simulink model "OA_Dynamic"  (R2020a)
settings: Solver=VariableStepAuto  StartTime=0.0  StopTime=30  RelTol=1e-3
values from neighbouring files (symbols this model uses):
  b = 0.4    [Takeoff.m]
  body_rate_0 = [0;0;0]    [Takeoff.m]
  Boundaries = [B1;B2;B3]    [Takeoff.m]
  Euler_0 = [0;0;0]    [Takeoff.m]
  g = [0;0;-9.8]    [Takeoff.m]
  I_Drone = [0.3933,0.3933,0.76]    [Takeoff.m]
  I_Tank = CalItank(m_tank,0.4,0.1,0.4,i)    [Takeoff.m]
  J = 0.00062    [Takeoff.m]
  K = 0.074    [Takeoff.m]
  k_T = MaxMotorThrsut/(MaxRPM^2)    (= 6.99167657551e-06)    [Takeoff.m]
  k_Thrsut2Torque = 0.021    [Takeoff.m]
  l = 0.5    [Takeoff.m]
  L = sqrt((x2-x1)^2 + (y2-y1)^2)    [Takeoff.m]
  m = m_drone + m_tank*percent    (= 36)    [Takeoff.m]    (also in animation.m = T_V1toI*T_V2toV1*T_BtoV2)
  m_drone = 20    [Takeoff.m]
  m_tank = 16    [Takeoff.m]
  MaxThrust = 4*MaxMotorThrsut    (= 529.2)    [Takeoff.m]
  MaxTilt = 30*pi/180    (= 0.523598775598)    [Takeoff.m]
  MaxTorque_XY = (T2-T1)*(l/sqrt(2))    [Takeoff.m]
  MaxVolt = 48    [Takeoff.m]
  MaxYawRate = 100*pi/180    (= 1.74532925199)    [Takeoff.m]
  MaxZVel = 2    [Takeoff.m]
  percent = 1    [Takeoff.m]
  Px1 = 0.2    [Takeoff.m]
  Pz1 = 1    [Takeoff.m]
  Pz2 = 100    [Takeoff.m]
  R = 0.0062    [Takeoff.m]
  RecObstacle = [[5,4,3] ... (first row only)    [Takeoff.m]
  SafeZone = 1.0    (= 1)    [Takeoff.m]
  Target = WayPts(3,:)    [Takeoff.m]
  ts = 0.01    [Takeoff.m]
  WayPts = [[XYZ_0(1) XYZ_0(2) XYZ_0(3)] ... (first row only)    [Takeoff.m]
  XYZ_0 = [0;0;0]    [Takeoff.m]
undefined symbols (not defined in the file or in its folder): b_tank, d_drone, d_tank, DiscIntNeverNeededParam, FlyVel, h_tank, PD1, PD2, PI1, PI2, PP1, PP2, SafeFactor, Sensor0Dir, TestVel
libraries: simulink x27, vrlib x4
(part 3 of 3)

== system OA_Dynamic/Controller/Rotors System/Propellers/Motor Thrust Control1/DC Motor ==
  note: d2/dt2(theta)
  note: d/dt(theta)
  note: d/dt(i)
  note: i
  Voltage : Inport
  TQ_load : Inport  Port=2
  Add : Sum  Inputs=-+-
  Add1 : Sum  Inputs=+--
  Damping : Gain  Gain=b
  Inductance : Gain  Gain=1/L
  Inertia : Gain  Gain=1/J
  Integrator : Integrator
  Integrator1 : Integrator
  Ke : Gain  Gain=K
  Kt : Gain  Gain=K
  Resistance : Gain  Gain=R
  Scope : Scope  NumInputPorts=2
  Speed : Outport
  wires:
  TQ_load/1 -> Add1/3
  Add1/1 -> Inertia/1
  Add/1 -> Inductance/1
  Ke/1 -> Add/3
  Damping/1 -> Add1/2
  Resistance/1 -> Add/1
  Voltage/1 -> Add/2
  Kt/1 -> Add1/1
  Integrator/1 -> Resistance/1, Scope/1, Kt/1
  Inertia/1 -> Integrator1/1
  Integrator1/1 -> Ke/1, Speed/1, Scope/2, Damping/1
  Inductance/1 -> Integrator/1

== system OA_Dynamic/Controller/Rotors System/Propellers/Motor Thrust Control2/DC Motor ==
  note: i
  note: d/dt(i)
  note: d/dt(theta)
  note: d2/dt2(theta)
  Voltage : Inport
  TQ_load : Inport  Port=2
  Add : Sum  Inputs=-+-
  Add1 : Sum  Inputs=+--
  Damping : Gain  Gain=b
  Inductance : Gain  Gain=1/L
  Inertia : Gain  Gain=1/J
  Integrator : Integrator
  Integrator1 : Integrator
  Ke : Gain  Gain=K
  Kt : Gain  Gain=K
  Resistance : Gain  Gain=R
  Scope : Scope  NumInputPorts=2
  Speed : Outport
  wires:
  Inductance/1 -> Integrator/1
  Integrator1/1 -> Damping/1, Scope/2, Speed/1, Ke/1
  Inertia/1 -> Integrator1/1
  Integrator/1 -> Kt/1, Scope/1, Resistance/1
  Kt/1 -> Add1/1
  Voltage/1 -> Add/2
  Resistance/1 -> Add/1
  Damping/1 -> Add1/2
  Ke/1 -> Add/3
  Add/1 -> Inductance/1
  Add1/1 -> Inertia/1
  TQ_load/1 -> Add1/3

== system OA_Dynamic/Controller/Rotors System/Propellers/Motor Thrust Control3/DC Motor ==
  note: d2/dt2(theta)
  note: d/dt(theta)
  note: d/dt(i)
  note: i
  Voltage : Inport
  TQ_load : Inport  Port=2
  Add : Sum  Inputs=-+-
  Add1 : Sum  Inputs=+--
  Damping : Gain  Gain=b
  Inductance : Gain  Gain=1/L
  Inertia : Gain  Gain=1/J
  Integrator : Integrator
  Integrator1 : Integrator
  Ke : Gain  Gain=K
  Kt : Gain  Gain=K
  Resistance : Gain  Gain=R
  Scope : Scope  NumInputPorts=2
  Speed : Outport
  wires:
  TQ_load/1 -> Add1/3
  Add1/1 -> Inertia/1
  Add/1 -> Inductance/1
  Ke/1 -> Add/3
  Damping/1 -> Add1/2
  Resistance/1 -> Add/1
  Voltage/1 -> Add/2
  Kt/1 -> Add1/1
  Integrator/1 -> Resistance/1, Scope/1, Kt/1
  Inertia/1 -> Integrator1/1
  Integrator1/1 -> Ke/1, Speed/1, Scope/2, Damping/1
  Inductance/1 -> Integrator/1

== matlab function OA_Dynamic/Controller/Sense X Y Distance/Sensor0 (30 degree sensor) ==
  data: Pos input; MinBDist output; Bounds input; Yaw input; MinBVect output; Directions input
function [MinBDist,MinBVect] = fcn(Pos,Bounds,Yaw,Directions)
MinBDist = 999;
MinBVect = [1;0;0];

for b = 1:size(Bounds,1)
Bound = Bounds(b,:);

%Bound = Bounds(BIndex,:);
MinSenseDist = 999;
MinSenseVect = [1;0;0];

for k = 1:size(Directions,2)
if length(Pos) > 1
    bx = Bound(1);
    by = Bound(2);
    tx = Bound(3);
    ty = Bound(4);
    X = Pos(1);
    Y = Pos(2);
    Z = Pos(3);
    
    m = [[cos(Yaw) -sin(Yaw)];[sin(Yaw) cos(Yaw)]];
    n = m*Directions(:,k); % Sense vector
    nx = n(1);
    ny = n(2);

    j = ((ty*bx-tx*by)-(ty*X-tx*Y))/(ty*nx-tx*ny);
    
    if j < 0 % sense backward point
        SenseDist = 999;
    else
        SensePt = [X+nx*j;Y+ny*j];
        
        % Check if ON boundaries
        if tx == 0
            i = (SensePt(2)-by)/ty;
        else
            i = (SensePt(1)-bx)/tx;
        end
        
        % If not
        if i < 0 || i > Bound(7)
            SenseDist = 999;
        % If yes
        else
            SenseDist = sqrt((nx*j)^2 + (ny*j)^2);
        end
    end
    
    SenseVect = [nx;ny;0]/sqrt(nx^2+ny^2);
    
else
    SenseDist = 999;
    SenseVect = [0;0;0];
end


if SenseDist < MinSenseDist
    MinSenseDist = SenseDist;
    MinSenseVect = SenseVect;
end
end

if MinSenseDist < MinBDist
    MinBDist = MinSenseDist;
    MinBVect = MinSenseVect;
end
end

== matlab function OA_Dynamic/6dof_system/Drone & Liquid Dynamic Inertia/DroneTankI ==
  data: I_D input; I output; I_T input; M_D input; M_T input; Z_D input; Z_T input; CR_X input; CR_Y input
function I = fcn(I_D,I_T,M_D,M_T,Z_D,Z_T,CR_X,CR_Y)

    Ix = I_D(1) + M_D*Z_D^2 + CR_X*I_T(1) + M_T*Z_T^2;
    Iy = I_D(2) + M_D*Z_D^2 + CR_Y*I_T(2) + M_T*Z_T^2;
    Iz = I_D(3) + I_T(3);
    I = [[Ix 0 0];[0 Iy 0];[0 0 Iz]];

== matlab function OA_Dynamic/6dof_system/Drone & Liquid Dynamic Inertia/FullTankCR ==
  data: w_d input; CR_x output; CR_y output; C_R input
function [CR_x,CR_y] = fcn(w_d,C_R)
if length(w_d) > 1
    if abs(w_d(2)) > 0.001
        CR_y = C_R;
    else
        CR_y = 1;
    end
    
    if abs(w_d(1)) > 0.001
        CR_x = C_R;
    else
        CR_x = 1;
    end
else
    CR_x = 1;
    CR_y = 1;
end

== matlab function OA_Dynamic/Controller/Subsystem1/MATLAB Function1 ==
  data: u input; y output
function y = fcn(u)
y = 0;
if u == 1
    y = 1;
end

== matlab function OA_Dynamic/Controller/Subsystem1/MATLAB Function2 ==
  data: u input; y output
function y = fcn(u)
y = 0;
if u == 3
    y = 1;
end

== matlab function OA_Dynamic/Controller/Rotors System/Motor2Drone ==
  data: FR input; Thrust output; Tq_R output; FL input; BR input; BL input; Tq_P output; Tq_Y output; l input; k input
function [Thrust,Tq_R,Tq_P,Tq_Y] = fcn(FR,FL,BR,BL,l,k)
% Tq_Y needs to change if using the real motor
    l_xy = l/sqrt(2);
    Thrust = FR + FL+ BR + BL;
    Tq_R = (FL+BL)*l_xy - (FR+BR)*l_xy;
    Tq_P = (BL+BR)*l_xy - (FL+FR)*l_xy;
    Tq_Y = (FR+BL)*k - (FL+BR)*k;

== matlab function OA_Dynamic/Controller/Rotors System/MotorThrustCmd ==
  data: Thrust_Cmd input; FR_Cmd output; FL_Cmd output; BR_Cmd output; BL_Cmd output; Tq_R_Cmd input; Tq_P_Cmd input; Tq_Y_Cmd input; l input; k input
function [FR_Cmd,FL_Cmd,BR_Cmd,BL_Cmd] = fcn(Thrust_Cmd,Tq_R_Cmd,Tq_P_Cmd,Tq_Y_Cmd,l,k)
    N = 4;
    l_xy = l/sqrt(2); % 45 degree configuration
    
    FR_Cmd = Thrust_Cmd/N + Tq_Y_Cmd/(N*k) - Tq_P_Cmd/(N*l_xy) - Tq_R_Cmd/(N*l_xy);
    FL_Cmd = Thrust_Cmd/N - Tq_Y_Cmd/(N*k) - Tq_P_Cmd/(N*l_xy) + Tq_R_Cmd/(N*l_xy);
    BR_Cmd = Thrust_Cmd/N - Tq_Y_Cmd/(N*k) + Tq_P_Cmd/(N*l_xy) - Tq_R_Cmd/(N*l_xy);
    BL_Cmd = Thrust_Cmd/N + Tq_Y_Cmd/(N*k) + Tq_P_Cmd/(N*l_xy) + Tq_R_Cmd/(N*l_xy);

== matlab function OA_Dynamic/Controller/Rotors System/Propellers/Motor Thrust Control/MATLAB Function ==
  data: u input; y output
function y = fcn(u)
    y = 0.000009*u^2;

    % The coefficient is decided by experimental value.
    % Max RPM = 4350, 48 Volt.

== matlab function OA_Dynamic/Controller/Rotors System/Propellers/Motor Thrust Control1/MATLAB Function ==
  data: u input; y output
function y = fcn(u)
    y = 0.000009*u^2;

    % The coefficient is decided by experimental value.
    % Max RPM = 4350, 48 Volt.

== matlab function OA_Dynamic/Controller/Rotors System/Propellers/Motor Thrust Control2/MATLAB Function ==
  data: u input; y output
function y = fcn(u)
    y = 0.000009*u^2;

    % The coefficient is decided by experimental value.
    % Max RPM = 4350, 48 Volt.

== matlab function OA_Dynamic/Controller/Rotors System/Propellers/Motor Thrust Control3/MATLAB Function ==
  data: u input; y output
function y = fcn(u)
    y = 0.000009*u^2;

    % The coefficient is decided by experimental value.
    % Max RPM = 4350, 48 Volt.

== matlab function OA_Dynamic/Select WayPoint/MATLAB Function ==
  data: WayPts input; CurrentWayPts output; WayPtsIndex input
function CurrentWayPts = fcn(WayPts,WayPtsIndex)
CurrentWayPts = WayPts(WayPtsIndex+1,:);

== matlab function OA_Dynamic/Select WayPoint/MATLAB Function1 ==
  data: CurrentWayPts input; TouchWayPts output; XYZ input; Index input; time input
function TouchWayPts = fcn(CurrentWayPts,XYZ,Index,time)
TouchWayPts = 0;

x = CurrentWayPts(1)-XYZ(1);
y = CurrentWayPts(2)-XYZ(2);
z = CurrentWayPts(3)-XYZ(3);
l = sqrt(x^2+y^2+z^2);

if Index == 0 && abs(l) < 0.1
    TouchWayPts = 1;
end

% if Index == 1 && abs(l) < 0.1
%     TouchWayPts = 1;
% end
if Index == 1 && time >= 10
    TouchWayPts = 1;
end

== matlab function OA_Dynamic/Controller/Sense Safe for Mode 2 and Mode 3 (count time based)/MATLAB Function1 ==
  data: mode input; IsTouchX input; count output; SenseX2 input
function count = fcn(mode,IsTouchX,SenseX2)
count = 0;
if mode == 1 && IsTouchX == 1 && SenseX2 > 100
    count = 1;
end

== matlab function OA_Dynamic/Controller/Sense Safe for Mode 2 and Mode 3 (count time based)/MATLAB Function2 ==
  data: mode input; IsTouchY input; count output; SenseY input
function count = fcn(mode,IsTouchY,SenseY)
count = 0;
if mode == 2 && IsTouchY == 1 && SenseY > 100
    count = 1;
end

== matlab function OA_Dynamic/Controller/Test For Decelerat Time/MATLAB Function3 ==
  data: time input; y output; XVel input
function y = fcn(time,XVel)
if time < 15
    y = 0;
else
    y = XVel;
end

== matlab function OA_Dynamic/Controller/Sense Safe for Mode 2 and Mode 3 (count time based)/MATLAB Function ==
  data: IsSensor0 input; count input; Vel input; BufferTime output; mode input; SafeZone input; SafeFactor input; DecelDist input; EdgeBuffer input
function BufferTime = fcn(IsSensor0,count,Vel,mode,SafeZone,SafeFactor,DecelDist,EdgeBuffer)

if mode == 1 && count == 1
% IsSensor0 will be 0 for the Case 1.
% For Case 2, Case 3, Add EdgeBuffer Time to guanrantee stability.
    if DecelDist < SafeZone
        if abs(Vel) >= 0.2
            BufferTime = SafeFactor*(SafeZone - DecelDist)/Vel + IsSensor0*EdgeBuffer;
        else
            BufferTime = 2;
        end
    else
        BufferTime = 0;
    end
    
else
    BufferTime = 2;
end

== matlab function OA_Dynamic/6dof_system/BtoITransform ==
  data: phi input; m output; theta input; psi input
function m = fcn(phi,theta,psi)
    T_BtoV2 = [[1 0 0];[0 cos(-phi) sin(-phi)];[0 -sin(-phi) cos(-phi)]];
    T_V2toV1 = [[cos(-theta) 0 -sin(-theta)];[0 1 0];[sin(-theta) 0 cos(-theta)]];
    T_V1toI = [[cos(-psi) sin(-psi) 0];[-sin(-psi) cos(-psi) 0];[0 0 1]];
    m = T_V1toI*T_V2toV1*T_BtoV2;

== matlab function OA_Dynamic/Controller/Sense X Y Distance/MATLAB Function ==
  data: mode input; Flag output; SenseY input
function Flag = fcn(mode,SenseY)
Flag = 0;
if mode == 2 && SenseY < 3
    Flag = 1;
end

== matlab function OA_Dynamic/Controller/Sense Safe for Mode 2 and Mode 3 (count time based)/MATLAB Function3 ==
  data: count input; Vel input; BufferTime output; mode input; SafeZone input; SafeFactor input; DecelDist input
function BufferTime = fcn(count,Vel,mode,SafeZone,SafeFactor,DecelDist)

if mode == 2 && count == 1
    if DecelDist < SafeZone
        if abs(Vel) >= 0.2
            BufferTime = SafeFactor*(SafeZone - DecelDist)/Vel;
        else
            BufferTime = 2;
        end
    else
        BufferTime = 0;
    end
else
    BufferTime = 2;
end

== matlab function OA_Dynamic/Controller/Sense Safe for Mode 2 and Mode 3 (count time based)/MATLAB Function4 ==
  data: mode input; Flag output; SenseX input; SafeZone input; SafeFactor input; IsSensorO input; DecelDist input
function Flag = fcn(mode,SenseX,SafeZone,SafeFactor,IsSensorO,DecelDist)
Flag = 0;

% SafeZone will increase to 1 if X distance is from Sensor0.

if mode == 0 && SenseX < (SafeZone + IsSensorO*0.5/sqrt(2)) + SafeFactor*DecelDist % SafeZone + SafeFactor * (Decel Distance)
    Flag = 1;
end

== matlab function OA_Dynamic/Controller/Sense X Y Distance/MATLAB Function1 ==
  data: Pos_SensorX1 output; l input; Pos input; Pos_SensorX2 output; Pos_SensorY1 output; m_BtoI input; Pos_SensorY2 output
function [Pos_SensorX1,Pos_SensorX2,Pos_SensorY1,Pos_SensorY2] = fcn(l,Pos,m_BtoI)
    X = Pos(1);
    Y = Pos(2);
    Z = Pos(3);
    
    % Sensor X1 Place
    Sx1_B = [1;0;0]+[0;-1;0];
    Sx1_B = Sx1_B/norm(Sx1_B);
    Sx1_B = l*Sx1_B;
    
    Sx1_I = m_BtoI*Sx1_B;
    Pos_SensorX1 = [X+Sx1_I(1);Y+Sx1_I(2);Z+Sx1_I(3)];
    
    
    % Sensor X2 Place
    Sx2_B = [1;0;0]+[0;1;0];
    Sx2_B = Sx2_B/norm(Sx2_B);
    Sx2_B = l*Sx2_B;
    
    Sx2_I = m_BtoI*Sx2_B;
    Pos_SensorX2 = [X+Sx2_I(1);Y+Sx2_I(2);Z+Sx2_I(3)];
    
    % Sensor Y1 Place
    Sy1_B = [-1;0;0]+[0;-1;0];
    Sy1_B = Sy1_B/norm(Sy1_B);
    Sy1_B = l*Sy1_B;
    
    Sy1_I = m_BtoI*Sy1_B;
    Pos_SensorY1 = [X+Sy1_I(1);Y+Sy1_I(2);Z+Sy1_I(3)];
    
    
    % Sensor Y2 Place
    Sy2_B = [-1;0;0]+[0;1;0];
    Sy2_B = Sy2_B/norm(Sy2_B);
    Sy2_B = l*Sy2_B;
    
    Sy2_I = m_BtoI*Sy2_B;
    Pos_SensorY2 = [X+Sy2_I(1);Y+Sy2_I(2);Z+Sy2_I(3)];

== matlab function OA_Dynamic/Controller/Sense Safe for Mode 2 and Mode 3 (count time based)/MATLAB Function5 ==
  data: mode input; count output; SenseX input; IsCrossOver input
function count = fcn(mode,SenseX,IsCrossOver)
count = 0;
if mode == 1 && IsCrossOver == true &&  SenseX > 100
    count = 1;
end

== matlab function OA_Dynamic/Controller/Sense X Y Distance/SensorY2 ==
  data: Pos input; MinSenseDist output; Bounds input; Yaw input; SenseVect output
function [MinSenseDist,SenseVect] = fcn(Pos,Bounds,Yaw)
MinSenseDist = 999;
for index = 1:size(Bounds,1)
    Bound = Bounds(index,:);
if length(Pos) > 1
    bx = Bound(1);
    by = Bound(2);
    tx = Bound(3);
    ty = Bound(4);
    X = Pos(1);
    Y = Pos(2);
    Z = Pos(3);
    
    m = [[cos(Yaw) -sin(Yaw)];[sin(Yaw) cos(Yaw)]];
    n = m*[0;1]; % Yb vector
    nx = n(1);
    ny = n(2);

    j = ((ty*bx-tx*by)-(ty*X-tx*Y))/(ty*nx-tx*ny);
    
    if j < 0 % sense backward point
        SenseDist = 999;
    else
        SensePt = [X+nx*j;Y+ny*j];
        
        % Check if ON boundaries
        if tx == 0
            i = (SensePt(2)-by)/ty;
        else
            i = (SensePt(1)-bx)/tx;
        end
        
        % If not
        if i < 0 || i > Bound(7)
            SenseDist = 999;
        % If yes
        else
            SenseDist = sqrt((nx*j)^2 + (ny*j)^2);
        end
    end
    
    SenseVect = [nx;ny;0];
    
else
    SenseDist = 999;
    SenseVect = [0;0;0];
end


if SenseDist < MinSenseDist
    MinSenseDist = SenseDist;
end


end

== matlab function OA_Dynamic/Controller/Sense X Y Distance/SensorX1 ==
  data: Pos input; MinSenseDist output; Bounds input; Yaw input; SenseVect output
function [MinSenseDist,SenseVect] = fcn(Pos,Bounds,Yaw)
MinSenseDist = 999;
for index = 1:size(Bounds,1)
    Bound = Bounds(index,:);
if length(Pos) > 1
    bx = Bound(1);
    by = Bound(2);
    tx = Bound(3);
    ty = Bound(4);
    X = Pos(1);
    Y = Pos(2);
    Z = Pos(3);
    
    m = [[cos(Yaw) -sin(Yaw)];[sin(Yaw) cos(Yaw)]];
    n = m*[1;0]; % Xb vector
    nx = n(1);
    ny = n(2);

    j = ((ty*bx-tx*by)-(ty*X-tx*Y))/(ty*nx-tx*ny);
    
    if j < 0 % sense backward point
        SenseDist = 999;
    else
        SensePt = [X+nx*j;Y+ny*j];
        
        % Check if ON boundaries
        if tx == 0
            i = (SensePt(2)-by)/ty;
        else
            i = (SensePt(1)-bx)/tx;
        end
        
        % If not
        if i < 0 || i > Bound(7)
            SenseDist = 999;
        % If yes
        else
            SenseDist = sqrt((nx*j)^2 + (ny*j)^2);
        end
    end
    
    SenseVect = [nx;ny;0];
    
else
    SenseDist = 999;
    SenseVect = [0;0;0];
end


if SenseDist < MinSenseDist
    MinSenseDist = SenseDist;
end


end

== matlab function OA_Dynamic/Controller/Sense X Y Distance/MATLAB Function3 ==
  data: mode input; SX1 input; NotSafe output; SX2 input; S0 input; S0Y input
function NotSafe = fcn(mode,SX1,SX2,S0,S0Y)
NotSafe = 0;
if mode == 0 && SX1 == 999 && SX2 == 999
    if S0 < 999
        if abs(S0Y) < 0.95
            NotSafe = 1;
        end
    end
end

== matlab function OA_Dynamic/Controller/Sense X Y Distance/SensorX2 ==
  data: Pos input; MinSenseDist output; Bounds input; Yaw input; SenseVect output
function [MinSenseDist,SenseVect] = fcn(Pos,Bounds,Yaw)
MinSenseDist = 999;
for index = 1:size(Bounds,1)
    Bound = Bounds(index,:);
if length(Pos) > 1
    bx = Bound(1);
    by = Bound(2);
    tx = Bound(3);
    ty = Bound(4);
    X = Pos(1);
    Y = Pos(2);
    Z = Pos(3);
    
    m = [[cos(Yaw) -sin(Yaw)];[sin(Yaw) cos(Yaw)]];
    n = m*[1;0]; % Xb vector
    nx = n(1);
    ny = n(2);

    j = ((ty*bx-tx*by)-(ty*X-tx*Y))/(ty*nx-tx*ny);
    
    if j < 0 % sense backward point
        SenseDist = 999;
    else
        SensePt = [X+nx*j;Y+ny*j];
        
        % Check if ON boundaries
        if tx == 0
            i = (SensePt(2)-by)/ty;
        else
            i = (SensePt(1)-bx)/tx;
        end
        
        % If not
        if i < 0 || i > Bound(7)
            SenseDist = 999;
        % If yes
        else
            SenseDist = sqrt((nx*j)^2 + (ny*j)^2);
        end
    end
    
    SenseVect = [nx;ny;0];
    
else
    SenseDist = 999;
    SenseVect = [0;0;0];
end


if SenseDist < MinSenseDist
    MinSenseDist = SenseDist;
end


end

== matlab function OA_Dynamic/6dof_system/euler_rate ==
  data: p input; phi_d output; q input; r input; phi input; theta input; theta_d output; psi_d output; psi input
function [phi_d,theta_d,psi_d] = fcn(p,q,r,phi,theta,psi)
    D = [[1 sin(phi)*tan(theta) cos(phi)*tan(theta)];
         [0 cos(phi) -sin(phi)];
         [0 sin(phi)/cos(theta) cos(phi)/cos(theta)]];
    euler_rate = D*[p;q;r]
    phi_d = euler_rate(1)
    theta_d = euler_rate(2)
    psi_d = euler_rate(3)

== matlab function OA_Dynamic/Force and Environment1/Floor Contact Force/MATLAB Function ==
  data: Thrust input; DetectTakeOff output; m input
function DetectTakeOff = fcn(Thrust,m)
DetectTakeOff = 0;
if Thrust >= m*9.8
    DetectTakeOff = 1;
end

== matlab function OA_Dynamic/Force and Environment1/Floor Contact Force/MATLAB Function1 ==
  data: IsTakeOff input; N output; Thrust input; m input
function N = fcn(IsTakeOff,Thrust,m)
if IsTakeOff == 0
    N = [0;0;m*9.8-Thrust];
else
    N = [0;0;0];
end

== matlab function OA_Dynamic/Controller/Sense X Y Distance/MATLAB Function6 ==
  data: mode input; SY output; SY1 input; SY2 input; Mode1Dir input
function SY = fcn(mode,SY1,SY2,Mode1Dir)
SY = 999;
if mode == 2
    if Mode1Dir == 1
        SY = SY2;
    else
        SY = SY1;
    end
end

== matlab function OA_Dynamic/Controller/Sense X Y Distance/SensorY1 ==
  data: Pos input; MinSenseDist output; Bounds input; Yaw input; SenseVect output
function [MinSenseDist,SenseVect] = fcn(Pos,Bounds,Yaw)
MinSenseDist = 999;
for index = 1:size(Bounds,1)
    Bound = Bounds(index,:);
if length(Pos) > 1
    bx = Bound(1);
    by = Bound(2);
    tx = Bound(3);
    ty = Bound(4);
    X = Pos(1);
    Y = Pos(2);
    Z = Pos(3);
    
    m = [[cos(Yaw) -sin(Yaw)];[sin(Yaw) cos(Yaw)]];
    n = m*[0;-1]; % Yb vector
    nx = n(1);
    ny = n(2);

    j = ((ty*bx-tx*by)-(ty*X-tx*Y))/(ty*nx-tx*ny);
    
    if j < 0 % sense backward point
        SenseDist = 999;
    else
        SensePt = [X+nx*j;Y+ny*j];
        
        % Check if ON boundaries
        if tx == 0
            i = (SensePt(2)-by)/ty;
        else
            i = (SensePt(1)-bx)/tx;
        end
        
        % If not
        if i < 0 || i > Bound(7)
            SenseDist = 999;
        % If yes
        else
            SenseDist = sqrt((nx*j)^2 + (ny*j)^2);
        end
    end
    
    SenseVect = [nx;ny;0];
    
else
    SenseDist = 999;
    SenseVect = [0;0;0];
end


if SenseDist < MinSenseDist
    MinSenseDist = SenseDist;
end


end

== matlab function OA_Dynamic/Controller/Sense X Y Distance/MATLAB Function8 ==
  data: u input; y output
function y = fcn(u)
if u >= 0
    y = 1;
else
    y = -1;
end

== matlab function OA_Dynamic/Controller/DynamicVelocity/MATLAB Function1 ==
  data: WaterLevel input; MaxVel output
function MaxVel = fcn(WaterLevel)
x = WaterLevel;

a = -0.0009323;
b = 6.146;
c = 1.17;
d = 0.01205;

MaxVel = a*exp(b*x) + c*exp(d*x);

== matlab function OA_Dynamic/Controller/MATLAB Function2 ==
  data: MaxVel input; Vx input; Vx_cal output; Vy input; Vy_cal output
function [Vx_cal,Vy_cal] = fcn(MaxVel,Vx,Vy)
if Vx > MaxVel
    Vx_cal = MaxVel;
elseif Vx < -MaxVel
    Vx_cal = -MaxVel;
else
    Vx_cal = Vx;
end

if Vy > MaxVel
    Vy_cal = MaxVel;
elseif Vy < -MaxVel
    Vy_cal = -MaxVel;
else
    Vy_cal = Vy;
end

== matlab function OA_Dynamic/Controller/Sense X Y Distance/MATLAB Function9 ==
  data: S0X output; l input; S0Y output; Vect input
function [S0X,S0Y] = fcn(l,Vect)
if length(Vect) > 1
    nx = Vect(1);
    ny = Vect(2);
    S0X = l*nx;
    S0Y = l*ny;
else
    S0Y = 0;
    S0X = 999;
end

== matlab function OA_Dynamic/Controller/Sense X Y Distance/MATLAB Function10 ==
  data: mode input; RightorLeft output; SX1 input; SX2 input; S0X input; S0Y input; IsSensor0 output; minSX input; SX output; Mode1Dir input; NotSafe input
function [RightorLeft,IsSensor0,SX] = fcn(mode,SX1,SX2,S0X,S0Y,minSX,Mode1Dir,NotSafe)
IsSensor0 = 0;
RightorLeft = 0;
SX = 999;
if mode == 0
    % First Case (Drone in the Boundaries)
    if SX1 < 100 && SX2 < 100
        % Decide Direction
        if SX1 >= SX2
            RightorLeft = 1;
        else
            RightorLeft = -1;
        end
        SX = minSX;

    % Second Case (Drone outside the Boundaries)    
    elseif SX1 == 999 && SX2 == 999 && S0X <= SX1
        IsSensor0 = 1;
        if S0Y >= 0
            RightorLeft = 1; 
        else
            RightorLeft = -1;
        end
        
        if NotSafe == true
            SX = S0X;
        else
            SX = 999;
        end
        
    % Third Case (Drone at the Edge of the Boundaries)
    elseif SX1 == 999 || SX2 == 999
        IsSensor0 = 1;
        if SX1 >= SX2
            RightorLeft = 1;
        else
            RightorLeft = -1;
        end
        SX = S0X;
    end   
end


if mode == 1
    if Mode1Dir >= 1
        SX = SX2;
    else
        SX = SX1;
    end
end

== matlab function OA_Dynamic/Controller/Sense X Y Distance/MATLAB Function5 ==
  data: mode input; flag output; SX input; S0Y input; SlowDownDist input; SlowBuffer input
function flag = fcn(mode,SX,S0Y,SlowDownDist,SlowBuffer)
flag = 0;
if mode == 0 && SX < SlowDownDist + SlowBuffer && abs(S0Y) < 0.95
    flag = 100;
end

if mode == 4
    flag = -100;
end

== matlab function OA_Dynamic/Controller/DynamicVelocity/MATLAB Function3 ==
  data: NeedAvoid input; Vel output; FlyVel input; MaxVel input
function Vel = fcn(NeedAvoid,FlyVel,MaxVel)
if NeedAvoid == 1
    Vel = MaxVel;
else
    Vel = FlyVel;
end

== matlab function OA_Dynamic/Controller/Sense X Y Distance/MATLAB Function7 ==
  data: Accel input; SlowDownDist output; Vx input
function SlowDownDist = fcn(Accel,Vx)
    SlowDownDist = 0.5*Vx^2/Accel;

== matlab function OA_Dynamic/Controller/Sense X Y Distance/MATLAB Function11 ==
  data: u input; y output
function y = fcn(u)
    y = 9.8*tan(u);

== matlab function OA_Dynamic/Controller/Test For Decelerat Time/MATLAB Function1 ==
  data: time input; count output; XVel input; stop output; IsZero input
function [count,stop] = fcn(time,XVel,IsZero)
stop = 0;
count = 0;
if time >= 15
    if abs(XVel) < 0.1
        count = 0;
        stop = 1;
    else
        if IsZero ~= true
            count = 1;
        end
    end
end

== matlab function OA_Dynamic/6dof_system/Drone & Liquid Dynamic Inertia/MATLAB Function ==
  data: hb_ratio input; C_R output
function C_R = fcn(hb_ratio)
x = hb_ratio;
p1 = -1.311;
p2 = 4.077;
p3 = -3.342;
p4 = -0.2563;
p5 = 0.9878;
C_R = p1*x^4 + p2*x^3 + p3*x^2 + p4*x + p5;

== matlab function OA_Dynamic/Controller/MATLAB Function ==
  data: Xe input; xb output; Ye input; psi input; yb output
function [xb,yb] = fcn(Xe,Ye,psi)
    m = [[cos(psi) sin(psi)];[-sin(psi) cos(psi)]]
    pos = m*[Xe;Ye]
    xb = pos(1)
    yb = pos(2)

== matlab function OA_Dynamic/Controller/Sense X Y Distance/MATLAB Function2 ==
  data: mode input; Flag output; SenseX2 input
function Flag = fcn(mode,SenseX2)
Flag = 0;
if mode == 1 && SenseX2 < 3
    Flag = 1;
end

== matlab function OA_Dynamic/6dof_system/ItoBTransform ==
  data: phi input; m output; theta input; psi input
function m = fcn(phi,theta,psi)
    T_ItoV1 = [[cos(psi) sin(psi) 0];[-sin(psi) cos(psi) 0];[0 0 1]]; 
    T_V1toV2 = [[cos(theta) 0 -sin(theta)];[0 1 0];[sin(theta) 0 cos(theta)]];
    T_V2toB = [[1 0 0];[0 cos(phi) sin(phi)];[0 -sin(phi) cos(phi)]];
    m = T_V2toB*T_V1toV2*T_ItoV1

== matlab function OA_Dynamic/WayPts to XYZerror ==
  data: waypts input; XYZerror output; XYZ input
function XYZerror = fcn(waypts,XYZ)
if length(waypts) > 1
    Xerror = waypts(1)-XYZ(1);
    Yerror = waypts(2)-XYZ(2);
    Zerror = waypts(3)-XYZ(3);
    XYZerror = [Xerror;Yerror;Zerror];
else
    XYZerror = [0;0;0];
end

== matlab function OA_Dynamic/Controller/ModeTrigger ==
  data: mode input; action output; IsSafe2Mode1 input; IsSafe2Mode2 input; IsSafe2Mode3 input; IsRecover input
function action = fcn(mode,IsSafe2Mode1,IsSafe2Mode2,IsSafe2Mode3,IsRecover)
action = 0;

% Approaching Mode
if mode == 0 && IsSafe2Mode1 == true 
   action = 1; % Stop Forward and Move Right
end

% Over Obstacle Mode
if mode == 1 && IsSafe2Mode2 == true 
    action = 1; % Stop Right and Move Forward
end
if mode == 2 && IsSafe2Mode3 == true
    action = 1; % Stop Forward and Move Left
end

%  Leaving Mode
if mode == 3 && IsRecover == 1
    action = 1; % Start to recover
end

== matlab function OA_Dynamic/Controller/ModeToCmd ==
  data: mode input; ForwardCmd output; YbVelCmd output; RefForward input; RefYbVel input; MaxVel input; Mode1Dir input
function [ForwardCmd,YbVelCmd] = fcn(mode,RefForward,RefYbVel,MaxVel,Mode1Dir)
ForwardCmd = RefForward;
YbVelCmd = RefYbVel;
if mode == 0
    ForwardCmd = RefForward;
    YbVelCmd = 0;    
elseif mode == 1
    ForwardCmd = 0;
    YbVelCmd = -Mode1Dir*MaxVel;
elseif mode == 2
    ForwardCmd = MaxVel;
    YbVelCmd = 0;
elseif mode == 3
    ForwardCmd = 0;
    YbVelCmd = (Mode1Dir)*MaxVel;
elseif mode > 3 
    ForwardCmd = MaxVel;
    YbVelCmd = RefYbVel;
end
